simulink model "Block_Diagram"  (R2026a)
settings: Solver=VariableStepAuto
values from neighbouring files (symbols this model uses):
  a_max = 27.4912    [PID.m]    (also in export_rod.m = j_max*t_j; end; optimize_trajectory.m = j_max * t_j; s_curve_cal.m = 27.49116213; simulate_cascade_pid_with_rod.m)
  B = 0.001    [create_simu.m]    (also in cross_validation.m = 0.19279; fix_plot_2.m = 0.19279; motor_grey_ode.m = [1/L_m; 0]; motor_grey_ode_v2.m = [1/L_m; 0])
  eta = 0.83607    [PID.m]    (also in create_simu.m = 0.85; cross_validation.m; export_rod.m; fix_plot_2.m)
  J = 0.72762    [PID.m]    (also in create_simu.m = 0.2546; cross_validation.m; export_rod.m; fix_plot_2.m)
  j_max = 1400.40    (= 1400.4)    [PID.m]    (also in export_rod.m = c.j_max; optimize_trajectory.m = x(3); s_curve_cal.m = 1400.3997989; simulate_cascade_pid_with_rod.m)
  K_e = 0.04165    [PID.m]    (also in create_simu.m = 0.0321; cross_validation.m; export_rod.m; fix_plot_2.m)
  K_t = 0.04065    [PID.m]    (also in create_simu.m = 0.0382; cross_validation.m; export_rod.m; fix_plot_2.m)
  L_m = 0.00144802    [PID.m]    (also in create_simu.m = 0.00147261; cross_validation.m; export_rod.m; fix_plot_2.m = 0.001448)
  N_total = 70    [PID.m]    (also in create_simu.m; cross_validation.m; export_rod.m; fix_plot_2.m)
  R_m = 1.45336    [PID.m]    (also in create_simu.m = 1.53982909; cross_validation.m = 1.45336105; export_rod.m; fix_plot_2.m = 1.4534)
  v_max = 7.3044    [PID.m]    (also in export_rod.m = c.v_max; optimize_trajectory.m = x(1); s_curve_cal.m = sqrt(a_max * q_total / 2 - a_max^2 / (2*j_max)); simulate_cascade_pid_with_rod.m)
undefined symbols (not defined in the file or in its folder): K_aff, K_vff, q_final, q_init
libraries: slpidlib x2, dspfdesign x1
settings Model: Creator=thadzy  LastModifiedBy=thadzy

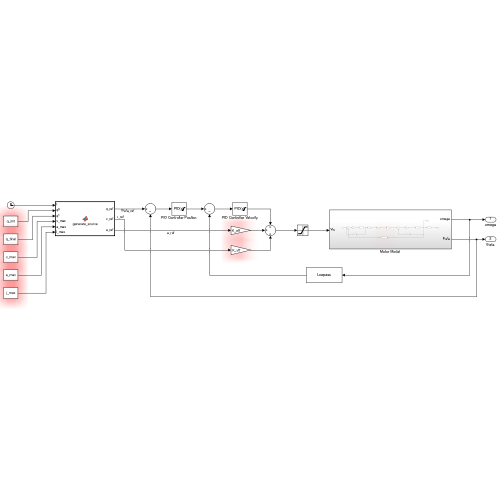
[thumbnail: Simulink's stored preview of the top-level diagram]
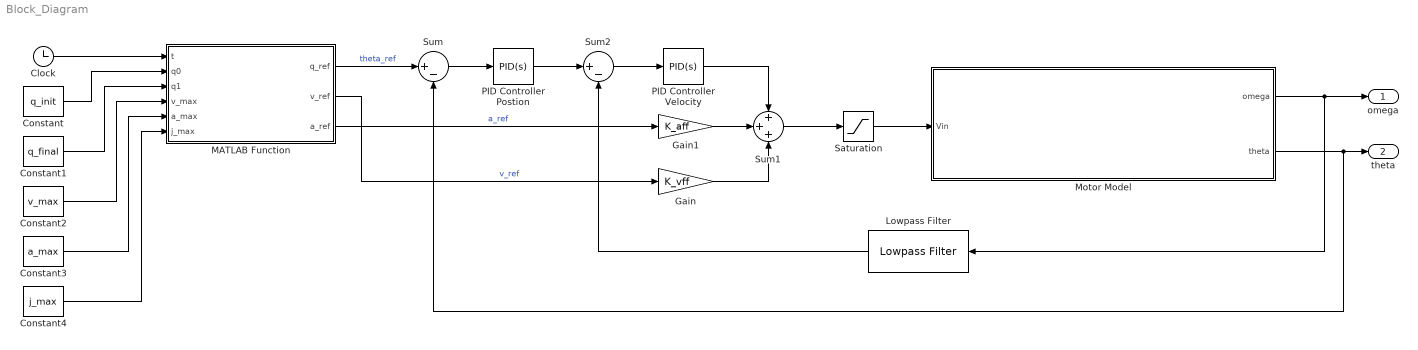
== system Block_Diagram ==
  Clock : Clock
  Constant : Constant  Value=q_init
  Constant1 : Constant  Value=q_final
  Constant2 : Constant  Value=v_max
  Constant3 : Constant  Value=a_max
  Constant4 : Constant  Value=j_max
  Gain : Gain  Gain=K_vff
  Gain1 : Gain  Gain=K_aff
  Lowpass Filter : dspfdesign/Lowpass Filter  FilterType=FIR  DesignForMinimumOrder=on  FilterOrder=50  PassbandFrequency=0.3628  StopbandFrequency=0.5442  PassbandRipple=0.1  StopbandAttenuation=80  SampleRateMode=Use normalized frequency (0 to 1)  SampleRate=44100  SimulateUsing=Interpreted execution  roundingMode=Floor  coeffsDataTypeStr=fixdt(1,16)
  MATLAB Function : MATLAB Function  TreatAsAtomicUnit=on
  Motor Model : Subsystem
  PID Controller Postion : slpidlib/PID Controller  Controller=PID  Form=Parallel  TimeDomain=Continuous-time  UseExternalTs=off  SampleTime=-1  IntegratorMethod=Forward Euler  FilterMethod=Forward Euler  ControllerParametersSource=internal  P=1  I=0  UseKiTs=off  D=0.5  UseExternalDerivativeSource=off  N=200  UseFilter=on  TunerSelectOption=Transfer Function Based (PID Tuner App)  InitialConditionSource=internal  InitialConditionForIntegrator=0  InitialConditionForFilter=0  DifferentiatorICPrevScaledInput=0  ExternalReset=none  TrackingMode=off  Kt=1  LimitOutput=on  SatLimitsSource=internal  UpperSaturationLimit=24  LowerSaturationLimit=-24  LinearizeAsGain=on  AntiWindupMode=clamping  Kb=1  LimitIntegrator=off  UpperIntegratorSaturationLimit=inf  LowerIntegratorSaturationLimit=-inf  POutMin=[]  POutMax=[]  IOutMin=[]  IOutMax=[]  DOutMin=[]  DOutMax=[]  NOutMin=[]  NOutMax=[]  SumOutMin=[]  SumOutMax=[]  SaturationOutMin=[]  SaturationOutMax=[]  PParamMin=[]  PParamMax=[]  IParamMin=[]  IParamMax=[]  DParamMin=[]  DParamMax=[]  NParamMin=[]  NParamMax=[]  KbParamMin=[]  KbParamMax=[]  KtParamMin=[]  KtParamMax=[]  KbOutMin=[]  KbOutMax=[]  KtOutMin=[]  KtOutMax=[]  IntegratorOutMin=[]  IntegratorOutMax=[]  FilterOutMin=[]  FilterOutMax=[]  SumI1OutMin=[]  SumI1OutMax=[]  SumI2OutMin=[]  SumI2OutMax=[]  SumI3OutMin=[]  SumI3OutMax=[]  SumI4OutMin=[]  SumI4OutMax=[]  SumDOutMin=[]  SumDOutMax=[]  DifferentiatorOutMin=[]  DifferentiatorOutMax=[]  FilterDiffOutCoefMin=[]  FilterDiffOutCoefMax=[]  ReciprocalOutMin=[]  ReciprocalOutMax=[]  SumDenOutMin=[]  SumDenOutMax=[]  SumNumOutMin=[]  SumNumOutMax=[]  DivideOutMin=[]  DivideOutMax=[]  UdiffTsProdOutMin=[]  UdiffTsProdOutMax=[]  NTsProdOutMin=[]  NTsProdOutMax=[]  UintegralTsProdOutMin=[]  UintegralTsProdOutMax=[]  UngainTsProdOutMin=[]  UngainTsProdOutMax=[]  ClampingZeroOutDataTypeStr=Inherit: Inherit via back propagation  ClampingZeroOutMin=[]  ClampingZeroOutMax=[]  FilterDenConstantOutDataTypeStr=Inherit: Inherit via back propagation  FilterDenConstantOutMin=[]  FilterDenConstantOutMax=[]  PCopyOutDataTypeStr=Inherit: Inherit via back propagation  PCopyOutMin=[]  PCopyOutMax=[]  NCopyOutDataTypeStr=Inherit: Inherit via back propagation  NCopyOutMin=[]  NCopyOutMax=[]  IntegratorContinuousStateAttributes=''  IntegratorStateMustResolveToSignalObject=off  IntegratorRTWStateStorageClass=Auto  FilterContinuousStateAttributes=''  FilterStateMustResolveToSignalObject=off  FilterRTWStateStorageClass=Auto  ParallelPVariant=InternalParameters  IdealPVariant=Disabled  IVariant=InternalParameters  DVariant=InternalParameters  IntegratorVariant=Continuous  SatVariant=Enabled  AWVariant=ContClampingParallel  PCopyVariant=Disabled  TRVariant=Disabled  FdbkBlocksVariant=Forward  IdealPFdbkVariant=Disabled  SatFdbkVariant=Disabled  DerivativeFilterVariant=ContFilter  NVariant=InternalParameters  NCopyVariant=Disabled  FilterICVariant=InternalICsFilter  IntegratorICVariant=InternalICs  ExternalResetVariant=Disabled  TRSumVariant=Passthrough  SumFdbkVariant=Disabled  SumVariant=Sum_PID  TsampFilterVariant=InternalTs  TsampNgainVariant=Passthrough  TsampIntegralVariant=Disabled_SignalSpec  ExternalSaturationOutDataTypeStr=Inherit: Same as second input  DerivativeSourceVariant=ErrorSignal  PreIntVariant=InternalPreInt
  PID Controller Velocity : slpidlib/PID Controller  Controller=PID  Form=Parallel  TimeDomain=Continuous-time  UseExternalTs=off  SampleTime=-1  IntegratorMethod=Forward Euler  FilterMethod=Forward Euler  ControllerParametersSource=internal  P=1  I=0  UseKiTs=off  D=0.5  UseExternalDerivativeSource=off  N=200  UseFilter=on  TunerSelectOption=Transfer Function Based (PID Tuner App)  InitialConditionSource=internal  InitialConditionForIntegrator=0  InitialConditionForFilter=0  DifferentiatorICPrevScaledInput=0  ExternalReset=none  TrackingMode=off  Kt=1  LimitOutput=on  SatLimitsSource=internal  UpperSaturationLimit=24  LowerSaturationLimit=-24  LinearizeAsGain=on  AntiWindupMode=clamping  Kb=1  LimitIntegrator=off  UpperIntegratorSaturationLimit=inf  LowerIntegratorSaturationLimit=-inf  POutMin=[]  POutMax=[]  IOutMin=[]  IOutMax=[]  DOutMin=[]  DOutMax=[]  NOutMin=[]  NOutMax=[]  SumOutMin=[]  SumOutMax=[]  SaturationOutMin=[]  SaturationOutMax=[]  PParamMin=[]  PParamMax=[]  IParamMin=[]  IParamMax=[]  DParamMin=[]  DParamMax=[]  NParamMin=[]  NParamMax=[]  KbParamMin=[]  KbParamMax=[]  KtParamMin=[]  KtParamMax=[]  KbOutMin=[]  KbOutMax=[]  KtOutMin=[]  KtOutMax=[]  IntegratorOutMin=[]  IntegratorOutMax=[]  FilterOutMin=[]  FilterOutMax=[]  SumI1OutMin=[]  SumI1OutMax=[]  SumI2OutMin=[]  SumI2OutMax=[]  SumI3OutMin=[]  SumI3OutMax=[]  SumI4OutMin=[]  SumI4OutMax=[]  SumDOutMin=[]  SumDOutMax=[]  DifferentiatorOutMin=[]  DifferentiatorOutMax=[]  FilterDiffOutCoefMin=[]  FilterDiffOutCoefMax=[]  ReciprocalOutMin=[]  ReciprocalOutMax=[]  SumDenOutMin=[]  SumDenOutMax=[]  SumNumOutMin=[]  SumNumOutMax=[]  DivideOutMin=[]  DivideOutMax=[]  UdiffTsProdOutMin=[]  UdiffTsProdOutMax=[]  NTsProdOutMin=[]  NTsProdOutMax=[]  UintegralTsProdOutMin=[]  UintegralTsProdOutMax=[]  UngainTsProdOutMin=[]  UngainTsProdOutMax=[]  ClampingZeroOutDataTypeStr=Inherit: Inherit via back propagation  ClampingZeroOutMin=[]  ClampingZeroOutMax=[]  FilterDenConstantOutDataTypeStr=Inherit: Inherit via back propagation  FilterDenConstantOutMin=[]  FilterDenConstantOutMax=[]  PCopyOutDataTypeStr=Inherit: Inherit via back propagation  PCopyOutMin=[]  PCopyOutMax=[]  NCopyOutDataTypeStr=Inherit: Inherit via back propagation  NCopyOutMin=[]  NCopyOutMax=[]  IntegratorContinuousStateAttributes=''  IntegratorStateMustResolveToSignalObject=off  IntegratorRTWStateStorageClass=Auto  FilterContinuousStateAttributes=''  FilterStateMustResolveToSignalObject=off  FilterRTWStateStorageClass=Auto  ParallelPVariant=InternalParameters  IdealPVariant=Disabled  IVariant=InternalParameters  DVariant=InternalParameters  IntegratorVariant=Continuous  SatVariant=Enabled  AWVariant=ContClampingParallel  PCopyVariant=Disabled  TRVariant=Disabled  FdbkBlocksVariant=Forward  IdealPFdbkVariant=Disabled  SatFdbkVariant=Disabled  DerivativeFilterVariant=ContFilter  NVariant=InternalParameters  NCopyVariant=Disabled  FilterICVariant=InternalICsFilter  IntegratorICVariant=InternalICs  ExternalResetVariant=Disabled  TRSumVariant=Passthrough  SumFdbkVariant=Disabled  SumVariant=Sum_PID  TsampFilterVariant=InternalTs  TsampNgainVariant=Passthrough  TsampIntegralVariant=Disabled_SignalSpec  ExternalSaturationOutDataTypeStr=Inherit: Same as second input  DerivativeSourceVariant=ErrorSignal  PreIntVariant=InternalPreInt
  Saturation : Saturate  UpperLimit=24  LowerLimit=-24
  Sum : Sum  Inputs=|+-
  Sum1 : Sum  Inputs=+++
  Sum2 : Sum  Inputs=|+-
  omega : Outport
  theta : Outport  Port=2
  wires:
  MATLAB Function/2(v_ref) -> Gain/1  "v_ref"
  Clock/1 -> MATLAB Function/1(t)
  Sum1/1 -> Saturation/1
  Gain/1 -> Sum1/3
  MATLAB Function/1(q_ref) -> Sum/1  "theta_ref"
  MATLAB Function/3(a_ref) -> Gain1/1  "a_ref"
  Gain1/1 -> Sum1/2
  Constant2/1 -> MATLAB Function/4(v_max)
  Sum/1 -> PID Controller Postion/1
  Constant/1 -> MATLAB Function/2(q0)
  Constant3/1 -> MATLAB Function/5(a_max)
  Constant1/1 -> MATLAB Function/3(q1)
  Constant4/1 -> MATLAB Function/6(j_max)
  PID Controller Postion/1 -> Sum2/1
  Sum2/1 -> PID Controller Velocity/1
  PID Controller Velocity/1 -> Sum1/1
  Motor Model/1(omega) -> omega/1, Lowpass Filter/1
  Saturation/1 -> Motor Model/1(Vin)
  Motor Model/2(theta) -> theta/1, Sum/2
  Lowpass Filter/1 -> Sum2/2

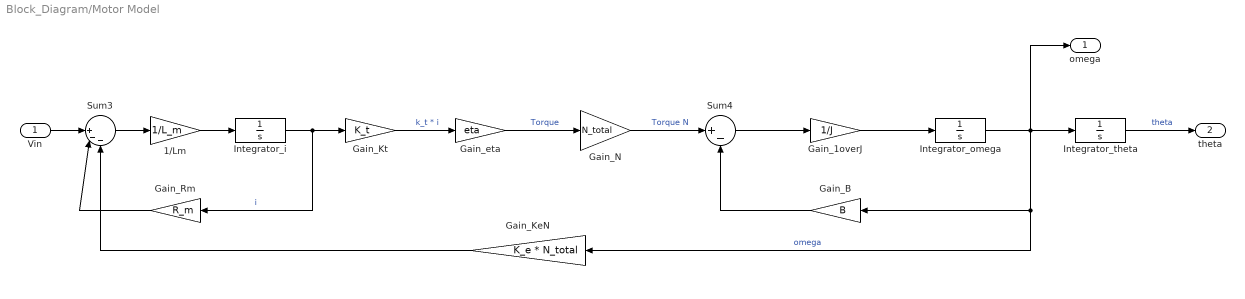
== system Block_Diagram/Motor Model ==
  Vin : Inport
  1/Lm : Gain  Gain=1/L_m
  Gain_1overJ : Gain  Gain=1/J
  Gain_B : Gain  Gain=B
  Gain_KeN : Gain  Gain=K_e * N_total
  Gain_Kt : Gain  Gain=K_t
  Gain_N : Gain  Gain=N_total
  Gain_Rm : Gain  Gain=R_m
  Gain_eta : Gain  Gain=eta
  Integrator_i : Integrator
  Integrator_omega : Integrator
  Integrator_theta : Integrator
  Sum3 : Sum  Inputs=||+--
  Sum4 : Sum  Inputs=|+-
  omega : Outport
  theta : Outport  Port=2
  wires:
  Gain_N/1 -> Sum4/1  "Torque N"
  Gain_B/1 -> Sum4/2
  1/Lm/1 -> Integrator_i/1
  Gain_1overJ/1 -> Integrator_omega/1
  Integrator_theta/1 -> theta/1  "theta"
  Gain_Kt/1 -> Gain_eta/1  "k_t * i"
  Integrator_omega/1 -> omega/1, Integrator_theta/1, Gain_KeN/1, Gain_B/1  "omega"
  Sum4/1 -> Gain_1overJ/1
  Sum3/1 -> 1/Lm/1
  Gain_KeN/1 -> Sum3/3
  Vin/1 -> Sum3/1
  Gain_Rm/1 -> Sum3/2
  Gain_eta/1 -> Gain_N/1  "Torque"
  Integrator_i/1 -> Gain_Kt/1, Gain_Rm/1  "i"

== matlab function Block_Diagram/MATLAB Function ==
  data: t input; q_ref output; q0 input; q1 input; v_max input; a_max input; j_max input; v_ref output; a_ref output
% /**
%  * @function generate_scurve
%  * @description Generates a complete 7-segment jerk-limited S-Curve trajectory.
%  * @param {double} t - Current simulation time (s).
%  * @param {double} q0 - Initial position (rad).
%  * @param {double} q1 - Final target position (rad).
%  * @param {double} v_max - Maximum allowable velocity (rad/s).
%  * @param {double} a_max - Maximum allowable acceleration (rad/s^2).
%  * @param {double} j_max - Maximum allowable jerk (rad/s^3).
%  * @returns {double} q_ref - Reference position at time t.
%  * @returns {double} v_ref - Reference velocity at time t.
%  * @returns {double} a_ref - Reference acceleration at time t.
%  */
function [q_ref, v_ref, a_ref] = generate_scurve(t, q0, q1, v_max, a_max, j_max)
    
    % Calculate total displacement and phase durations
    h = q1 - q0;
    tj = a_max / j_max;
    ta = v_max / a_max;
    tv = (h / v_max) - ta;
    
    % Time breakpoints
    t1 = tj;
    t2 = ta;
    t3 = ta + tj;
    t4 = ta + tj + tv;
    t7 = t4 + ta + tj; % Total trajectory time
    
    % Initial conditions
    if t <= 0
        q_ref = q0; v_ref = 0; a_ref = 0;
        
    % Acceleration Phase (Segments 1 to 3)
    elseif t < t1
        % Segment 1: Jerk bounded acceleration
        a_ref = j_max * t;
        v_ref = 0.5 * j_max * t^2;
        q_ref = q0 + (1/6) * j_max * t^3;
        
    elseif t < t2
        % Segment 2: Constant acceleration
        dt = t - t1;
        a_ref = a_max;
        v_ref = (0.5 * j_max * t1^2) + a_max * dt;
        q_ref = q0 + (1/6) * j_max * t1^3 + (0.5 * j_max * t1^2) * dt + 0.5 * a_max * dt^2;
        
    elseif t < t3
        % Segment 3: Jerk bounded deceleration to reach constant velocity
        dt = t - t2;
        a_ref = a_max - j_max * dt;
        v2 = (0.5 * j_max * t1^2) + a_max * (t2 - t1);
        q2 = q0 + (1/6) * j_max * t1^3 + (0.5 * j_max * t1^2) * (t2 - t1) + 0.5 * a_max * (t2 - t1)^2;
        v_ref = v2 + a_max * dt - 0.5 * j_max * dt^2;
        q_ref = q2 + v2 * dt + 0.5 * a_max * dt^2 - (1/6) * j_max * dt^3;
        
    % Constant Velocity Phase (Segment 4)
    elseif t < t4
        dt = t - t3;
        a_ref = 0;
        v_ref = v_max;
        q3 = q0 + h/2 - v_max * (tv/2);
        q_ref = q3 + v_max * dt;
        
    % Deceleration Phase using time-reversal symmetry (Segments 5 to 7)
    elseif t < t7
        tau = t7 - t; % Time remaining
        
        if tau < t1
            % Equivalent to Segment 7
            a_ref = -j_max * tau;
            v_ref = 0.5 * j_max * tau^2;
            q_ref = q1 - (1/6) * j_max * tau^3;
            
        elseif tau < t2
            % Equivalent to Segment 6
            dt_tau = tau - t1;
            a_ref = -a_max;
            v_ref = (0.5 * j_max * t1^2) + a_max * dt_tau;
            q_ref = q1 - ((1/6) * j_max * t1^3 + (0.5 * j_max * t1^2) * dt_tau + 0.5 * a_max * dt_tau^2);
            
        else
            % Equivalent to Segment 5
            dt_tau = tau - t2;
            a_ref = -a_max + j_max * dt_tau;
            v2_tau = (0.5 * j_max * t1^2) + a_max * (t2 - t1);
            q2_tau = (1/6) * j_max * t1^3 + (0.5 * j_max * t1^2) * (t2 - t1) + 0.5 * a_max * (t2 - t1)^2;
            v_ref = v2_tau + a_max * dt_tau - 0.5 * j_max * dt_tau^2;
            q_ref = q1 - (q2_tau + v2_tau * dt_tau + 0.5 * a_max * dt_tau^2 - (1/6) * j_max * dt_tau^3);
        end
        
    % Final State Reached
    else
        q_ref = q1;
        v_ref = 0;
        a_ref = 0;
    end
end
